simulink library "halout"  (R2021b)
settings: Solver=VariableStepAuto  StartTime=0.0  StopTime=10.0  RelTol=1e-3
undefined symbols (not defined in the file): C_TASK_5MS_S, FALSE, KHAL_CAN1FDAPS3E2E_flg, KHAL_CAN1FDAPS3TxReq_flg, KHAL_CAN1FDVCU2E2E_flg, KHAL_CAN1FDVCU2TxReq_flg, KHAL_CAN1FDVCU3E2E_flg, KHAL_CAN1FDVCU3TxReq_flg, KHAL_CAN1TxReq_flg, KHAL_CAN2TxReq_flg, KHAL_CAN3FDVCU1TxReq_flg, KHAL_CAN3FDVCU2E2E_flg, KHAL_CAN3FDVCU2TxReq_flg, KHAL_CAN3TxReq_flg, KHAL_CAN4FDVCU1E2E_flg, KHAL_CAN4FDVCU1TxReq_flg, KHAL_CAN4TxReq_flg, KHAL_CAN5TxReq_flg, ONE_INT, TRUE, ZERO_INT
libraries: FVT_lib x383, simulink x179
(part 6 of 20)

== system halout/HAL_OUT/CAN2/FD_VCU5_0x245 ==
  BSCP_outputs : Inport  OutDataTypeStr=Bus: BSCP_outputs
  BOUTP_outputs : Inport  Port=2  OutDataTypeStr=Bus: BOUTP_outputs
  EDriveSysErrAccPedalErr : Subsystem
  EDriveSysErrMCUErr : Subsystem
  EDriveSysErrShifterErr : Subsystem
  EDriveSysErrVCUErr : Subsystem
  Ground{,1..6} (7 alike) : Ground
  HVSysErrIsolationErr : Subsystem
  HVSysErrPackErr : Subsystem
  HVSysErrRelayErr : Subsystem
  LVSysErrPwrOutpErr : Subsystem
  LimphomeAct : Subsystem
  LowSOCWarn : Subsystem
  PwrStaErr : Subsystem
  ReVehThdChkSta : Subsystem
  bus_creator : BusCreator  Inputs=12  OutDataTypeStr=Bus: DT_CAN2_SG_FD_VCU5  NonVirtualBus=on
  bus_selector : BusSelector  OutputSignals=VOUTP_EDriveSysErr_VCUErrTmp_flg
  bus_selector1 : BusSelector  OutputSignals=VOUTP_LVSysErrPwrOutErr_flg
  bus_selector2 : BusSelector  OutputSignals=VOUTP_LimpHomeActTmp_flg
  bus_selector3 : BusSelector  OutputSignals=VOUTP_LowSOCWarn_enum
  bus_selector4 : BusSelector  OutputSignals=VOUTP_ReVehThdChkSta_enum
  FD_VCU5 : Outport
  wires:
  BSCP_outputs/1 -> [BSCP_outputs]
  BOUTP_outputs/1 -> [BOUTP_outputs]
  [CAN2_EDriveSysErr_AccPedalErr] -> bus_creator/1  "CAN2_EDriveSysErr_AccPedalErr"
  [CAN2_EDriveSysErr_MCUErr] -> bus_creator/2  "CAN2_EDriveSysErr_MCUErr"
  [CAN2_EDriveSysErr_ShifterErr] -> bus_creator/3  "CAN2_EDriveSysErr_ShifterErr"
  [CAN2_EDriveSysErr_VCUErr] -> bus_creator/4  "CAN2_EDriveSysErr_VCUErr"
  [CAN2_HVSysErr_IsolationErr] -> bus_creator/5  "CAN2_HVSysErr_IsolationErr"
  [CAN2_HVSysErr_PackErr] -> bus_creator/6  "CAN2_HVSysErr_PackErr"
  [CAN2_HVSysErr_RelayErr] -> bus_creator/7  "CAN2_HVSysErr_RelayErr"
  [CAN2_LVSysErr_PwrOutpErr] -> bus_creator/8  "CAN2_LVSysErr_PwrOutpErr"
  [CAN2_LimphomeAct] -> bus_creator/9  "CAN2_LimphomeAct"
  [CAN2_LowSOCWarn] -> bus_creator/10  "CAN2_LowSOCWarn"
  [CAN2_PwrStaErr] -> bus_creator/11  "CAN2_PwrStaErr"
  [CAN2_Re_VehThdChkSta] -> bus_creator/12  "CAN2_Re_VehThdChkSta"
  bus_creator/1 -> FD_VCU5/1
  EDriveSysErrAccPedalErr/1(CAN2_EDriveSysErr_AccPedalErr) -> [CAN2_EDriveSysErr_AccPedalErr]
  EDriveSysErrMCUErr/1(CAN2_EDriveSysErr_MCUErr) -> [CAN2_EDriveSysErr_MCUErr]
  EDriveSysErrShifterErr/1(CAN2_EDriveSysErr_ShifterErr) -> [CAN2_EDriveSysErr_ShifterErr]
  EDriveSysErrVCUErr/1(CAN2_EDriveSysErr_VCUErr) -> [CAN2_EDriveSysErr_VCUErr]
  HVSysErrIsolationErr/1(CAN2_HVSysErr_IsolationErr) -> [CAN2_HVSysErr_IsolationErr]
  HVSysErrPackErr/1(CAN2_HVSysErr_PackErr) -> [CAN2_HVSysErr_PackErr]
  HVSysErrRelayErr/1(CAN2_HVSysErr_RelayErr) -> [CAN2_HVSysErr_RelayErr]
  LVSysErrPwrOutpErr/1(CAN2_LVSysErr_PwrOutpErr) -> [CAN2_LVSysErr_PwrOutpErr]
  LimphomeAct/1(CAN2_LimphomeAct) -> [CAN2_LimphomeAct]
  LowSOCWarn/1(CAN2_LowSOCWarn) -> [CAN2_LowSOCWarn]
  PwrStaErr/1(CAN2_PwrStaErr) -> [CAN2_PwrStaErr]
  ReVehThdChkSta/1(CAN2_Re_VehThdChkSta) -> [CAN2_Re_VehThdChkSta]
  Ground/1 -> EDriveSysErrAccPedalErr/1(EDriveSysErrAccPedalErr)
  Ground1/1 -> EDriveSysErrMCUErr/1(EDriveSysErrMCUErr)
  Ground2/1 -> EDriveSysErrShifterErr/1(EDriveSysErrShifterErr)
  bus_selector/1 -> EDriveSysErrVCUErr/1(EDriveSysErrVCUErr)  "<VOUTP_EDriveSysErr_VCUErrTmp_flg>"
  [BOUTP_outputs] -> bus_selector/1
  Ground3/1 -> HVSysErrIsolationErr/1(HVSysErrIsolationErr)
  Ground4/1 -> HVSysErrPackErr/1(HVSysErrPackErr)
  Ground5/1 -> HVSysErrRelayErr/1(HVSysErrRelayErr)
  bus_selector1/1 -> LVSysErrPwrOutpErr/1(LVSysErrPwrOutpErr)  "<VOUTP_LVSysErrPwrOutErr_flg>"
  [BOUTP_outputs] -> bus_selector1/1
  bus_selector2/1 -> LimphomeAct/1(LimphomeAct)  "<VOUTP_LimpHomeActTmp_flg>"
  [BOUTP_outputs] -> bus_selector2/1
  bus_selector3/1 -> LowSOCWarn/1(LowSOCWarn)  "<VOUTP_LowSOCWarn_enum>"
  [BOUTP_outputs] -> bus_selector3/1
  Ground6/1 -> PwrStaErr/1(PwrStaErr)
  bus_selector4/1 -> ReVehThdChkSta/1(ReVehThdChkSta)  "<VOUTP_ReVehThdChkSta_enum>"
  [BOUTP_outputs] -> bus_selector4/1

== system halout/HAL_OUT/CAN2/FD_VCU6_0x3C3 ==
  BSCP_outputs : Inport  OutDataTypeStr=Bus: BSCP_outputs
  BOUTP_outputs : Inport  Port=2  OutDataTypeStr=Bus: BOUTP_outputs
  FUSIONHWVer1 : Subsystem
  FUSIONHWVer2 : Subsystem
  FUSIONHWVer3 : Subsystem
  FUSIONSWCarModel1 : Subsystem
  FUSIONSWCarModel2 : Subsystem
  FUSIONSWCarModel3 : Subsystem
  FUSIONSWController1 : Subsystem
  FUSIONSWController2 : Subsystem
  FUSIONSWCountry1 : Subsystem
  FUSIONSWCountry2 : Subsystem
  FUSIONSWMajor1 : Subsystem
  FUSIONSWMajor2 : Subsystem
  FUSIONSWMinor1 : Subsystem
  FUSIONSWMinor2 : Subsystem
  FUSIONSWPatch1 : Subsystem
  FUSIONSWPatch2 : Subsystem
  FUSIONSWSHA1 : Subsystem
  FUSIONSWSHA2 : Subsystem
  FUSIONSWSHA3 : Subsystem
  FUSIONSWSHA4 : Subsystem
  FUSIONSWSHA5 : Subsystem
  FUSIONSWSHA6 : Subsystem
  FUSIONSWSHA7 : Subsystem
  FUSIONSWSHA8 : Subsystem
  FUSIONSWVar : Subsystem
  FUSIONSWchange1 : Subsystem
  FUSIONSWchange2 : Subsystem
  FUSIONSWdash1 : Subsystem
  FUSIONSWdash2 : Subsystem
  bus_creator : BusCreator  Inputs=29  OutDataTypeStr=Bus: DT_CAN2_SG_FD_VCU6  NonVirtualBus=on
  bus_selector : BusSelector  OutputSignals=VOUTP_HWVer1_cnt
  bus_selector1 : BusSelector  OutputSignals=VOUTP_HWVer2_cnt
  bus_selector10 : BusSelector  OutputSignals=VOUTP_Major1_cnt
  bus_selector11 : BusSelector  OutputSignals=VOUTP_Major2_cnt
  bus_selector12 : BusSelector  OutputSignals=VOUTP_Minor1_cnt
  bus_selector13 : BusSelector  OutputSignals=VOUTP_Minor2_cnt
  bus_selector14 : BusSelector  OutputSignals=VOUTP_Patch1_cnt
  bus_selector15 : BusSelector  OutputSignals=VOUTP_Patch2_cnt
  bus_selector16 : BusSelector  OutputSignals=VOUTP_SHA1_cnt
  bus_selector17 : BusSelector  OutputSignals=VOUTP_SHA2_cnt
  bus_selector18 : BusSelector  OutputSignals=VOUTP_SHA3_cnt
  bus_selector19 : BusSelector  OutputSignals=VOUTP_SHA4_cnt
  bus_selector2 : BusSelector  OutputSignals=VOUTP_HWVer3_cnt
  bus_selector20 : BusSelector  OutputSignals=VOUTP_SHA5_cnt
  bus_selector21 : BusSelector  OutputSignals=VOUTP_SHA6_cnt
  bus_selector22 : BusSelector  OutputSignals=VOUTP_SHA7_cnt
  bus_selector23 : BusSelector  OutputSignals=VOUTP_SHA8_cnt
  bus_selector24 : BusSelector  OutputSignals=VOUTP_Variation_cnt
  bus_selector25 : BusSelector  OutputSignals=VOUTP_Change1_cnt
  bus_selector26 : BusSelector  OutputSignals=VOUTP_Change2_cnt
  bus_selector27 : BusSelector  OutputSignals=VOUTP_Dash1_cnt
  bus_selector28 : BusSelector  OutputSignals=VOUTP_Dash2_cnt
  bus_selector3 : BusSelector  OutputSignals=VOUTP_CarModel1_cnt
  bus_selector4 : BusSelector  OutputSignals=VOUTP_CarModel2_cnt
  bus_selector5 : BusSelector  OutputSignals=VOUTP_CarModel3_cnt
  bus_selector6 : BusSelector  OutputSignals=VOUTP_ECU1_cnt
  bus_selector7 : BusSelector  OutputSignals=VOUTP_ECU2_cnt
  bus_selector8 : BusSelector  OutputSignals=VOUTP_Country1_cnt
  bus_selector9 : BusSelector  OutputSignals=VOUTP_Country2_cnt
  FD_VCU6 : Outport
  wires:
  BSCP_outputs/1 -> [BSCP_outputs]
  BOUTP_outputs/1 -> [BOUTP_outputs]
  [CAN2_FUSION_HW_Ver1] -> bus_creator/1  "CAN2_FUSION_HW_Ver1"
  [CAN2_FUSION_HW_Ver2] -> bus_creator/2  "CAN2_FUSION_HW_Ver2"
  [CAN2_FUSION_HW_Ver3] -> bus_creator/3  "CAN2_FUSION_HW_Ver3"
  [CAN2_FUSION_SW_CarModel1] -> bus_creator/4  "CAN2_FUSION_SW_CarModel1"
  [CAN2_FUSION_SW_CarModel2] -> bus_creator/5  "CAN2_FUSION_SW_CarModel2"
  [CAN2_FUSION_SW_CarModel3] -> bus_creator/6  "CAN2_FUSION_SW_CarModel3"
  [CAN2_FUSION_SW_Controller1] -> bus_creator/7  "CAN2_FUSION_SW_Controller1"
  [CAN2_FUSION_SW_Controller2] -> bus_creator/8  "CAN2_FUSION_SW_Controller2"
  [CAN2_FUSION_SW_Country1] -> bus_creator/9  "CAN2_FUSION_SW_Country1"
  [CAN2_FUSION_SW_Country2] -> bus_creator/10  "CAN2_FUSION_SW_Country2"
  [CAN2_FUSION_SW_Major1] -> bus_creator/11  "CAN2_FUSION_SW_Major1"
  [CAN2_FUSION_SW_Major2] -> bus_creator/12  "CAN2_FUSION_SW_Major2"
  [CAN2_FUSION_SW_Minor1] -> bus_creator/13  "CAN2_FUSION_SW_Minor1"
  [CAN2_FUSION_SW_Minor2] -> bus_creator/14  "CAN2_FUSION_SW_Minor2"
  [CAN2_FUSION_SW_Patch1] -> bus_creator/15  "CAN2_FUSION_SW_Patch1"
  [CAN2_FUSION_SW_Patch2] -> bus_creator/16  "CAN2_FUSION_SW_Patch2"
  [CAN2_FUSION_SW_SHA1] -> bus_creator/17  "CAN2_FUSION_SW_SHA1"
  [CAN2_FUSION_SW_SHA2] -> bus_creator/18  "CAN2_FUSION_SW_SHA2"
  [CAN2_FUSION_SW_SHA3] -> bus_creator/19  "CAN2_FUSION_SW_SHA3"
  [CAN2_FUSION_SW_SHA4] -> bus_creator/20  "CAN2_FUSION_SW_SHA4"
  [CAN2_FUSION_SW_SHA5] -> bus_creator/21  "CAN2_FUSION_SW_SHA5"
  [CAN2_FUSION_SW_SHA6] -> bus_creator/22  "CAN2_FUSION_SW_SHA6"
  [CAN2_FUSION_SW_SHA7] -> bus_creator/23  "CAN2_FUSION_SW_SHA7"
  [CAN2_FUSION_SW_SHA8] -> bus_creator/24  "CAN2_FUSION_SW_SHA8"
  [CAN2_FUSION_SW_Var] -> bus_creator/25  "CAN2_FUSION_SW_Var"
  [CAN2_FUSION_SW_change1] -> bus_creator/26  "CAN2_FUSION_SW_change1"
  [CAN2_FUSION_SW_change2] -> bus_creator/27  "CAN2_FUSION_SW_change2"
  [CAN2_FUSION_SW_dash1] -> bus_creator/28  "CAN2_FUSION_SW_dash1"
  [CAN2_FUSION_SW_dash2] -> bus_creator/29  "CAN2_FUSION_SW_dash2"
  bus_creator/1 -> FD_VCU6/1
  FUSIONHWVer1/1(CAN2_FUSION_HW_Ver1) -> [CAN2_FUSION_HW_Ver1]
  FUSIONHWVer2/1(CAN2_FUSION_HW_Ver2) -> [CAN2_FUSION_HW_Ver2]
  FUSIONHWVer3/1(CAN2_FUSION_HW_Ver3) -> [CAN2_FUSION_HW_Ver3]
  FUSIONSWCarModel1/1(CAN2_FUSION_SW_CarModel1) -> [CAN2_FUSION_SW_CarModel1]
  FUSIONSWCarModel2/1(CAN2_FUSION_SW_CarModel2) -> [CAN2_FUSION_SW_CarModel2]
  FUSIONSWCarModel3/1(CAN2_FUSION_SW_CarModel3) -> [CAN2_FUSION_SW_CarModel3]
  FUSIONSWController1/1(CAN2_FUSION_SW_Controller1) -> [CAN2_FUSION_SW_Controller1]
  FUSIONSWController2/1(CAN2_FUSION_SW_Controller2) -> [CAN2_FUSION_SW_Controller2]
  FUSIONSWCountry1/1(CAN2_FUSION_SW_Country1) -> [CAN2_FUSION_SW_Country1]
  FUSIONSWCountry2/1(CAN2_FUSION_SW_Country2) -> [CAN2_FUSION_SW_Country2]
  FUSIONSWMajor1/1(CAN2_FUSION_SW_Major1) -> [CAN2_FUSION_SW_Major1]
  FUSIONSWMajor2/1(CAN2_FUSION_SW_Major2) -> [CAN2_FUSION_SW_Major2]
  FUSIONSWMinor1/1(CAN2_FUSION_SW_Minor1) -> [CAN2_FUSION_SW_Minor1]
  FUSIONSWMinor2/1(CAN2_FUSION_SW_Minor2) -> [CAN2_FUSION_SW_Minor2]
  FUSIONSWPatch1/1(CAN2_FUSION_SW_Patch1) -> [CAN2_FUSION_SW_Patch1]
  FUSIONSWPatch2/1(CAN2_FUSION_SW_Patch2) -> [CAN2_FUSION_SW_Patch2]
  FUSIONSWSHA1/1(CAN2_FUSION_SW_SHA1) -> [CAN2_FUSION_SW_SHA1]
  FUSIONSWSHA2/1(CAN2_FUSION_SW_SHA2) -> [CAN2_FUSION_SW_SHA2]
  FUSIONSWSHA3/1(CAN2_FUSION_SW_SHA3) -> [CAN2_FUSION_SW_SHA3]
  FUSIONSWSHA4/1(CAN2_FUSION_SW_SHA4) -> [CAN2_FUSION_SW_SHA4]
  FUSIONSWSHA5/1(CAN2_FUSION_SW_SHA5) -> [CAN2_FUSION_SW_SHA5]
  FUSIONSWSHA6/1(CAN2_FUSION_SW_SHA6) -> [CAN2_FUSION_SW_SHA6]
  FUSIONSWSHA7/1(CAN2_FUSION_SW_SHA7) -> [CAN2_FUSION_SW_SHA7]
  FUSIONSWSHA8/1(CAN2_FUSION_SW_SHA8) -> [CAN2_FUSION_SW_SHA8]
  FUSIONSWVar/1(CAN2_FUSION_SW_Var) -> [CAN2_FUSION_SW_Var]
  FUSIONSWchange1/1(CAN2_FUSION_SW_change1) -> [CAN2_FUSION_SW_change1]
  FUSIONSWchange2/1(CAN2_FUSION_SW_change2) -> [CAN2_FUSION_SW_change2]
  FUSIONSWdash1/1(CAN2_FUSION_SW_dash1) -> [CAN2_FUSION_SW_dash1]
  FUSIONSWdash2/1(CAN2_FUSION_SW_dash2) -> [CAN2_FUSION_SW_dash2]
  bus_selector/1 -> FUSIONHWVer1/1(FUSIONHWVer1)  "<VOUTP_HWVer1_cnt>"
  [BOUTP_outputs] -> bus_selector/1
  bus_selector1/1 -> FUSIONHWVer2/1(FUSIONHWVer2)  "<VOUTP_HWVer2_cnt>"
  [BOUTP_outputs] -> bus_selector1/1
  bus_selector2/1 -> FUSIONHWVer3/1(FUSIONHWVer3)  "<VOUTP_HWVer3_cnt>"
  [BOUTP_outputs] -> bus_selector2/1
  bus_selector3/1 -> FUSIONSWCarModel1/1(FUSIONSWCarModel1)  "<VOUTP_CarModel1_cnt>"
  [BOUTP_outputs] -> bus_selector3/1
  bus_selector4/1 -> FUSIONSWCarModel2/1(FUSIONSWCarModel2)  "<VOUTP_CarModel2_cnt>"
  [BOUTP_outputs] -> bus_selector4/1
  bus_selector5/1 -> FUSIONSWCarModel3/1(FUSIONSWCarModel3)  "<VOUTP_CarModel3_cnt>"
  [BOUTP_outputs] -> bus_selector5/1
  bus_selector6/1 -> FUSIONSWController1/1(FUSIONSWController1)  "<VOUTP_ECU1_cnt>"
  [BOUTP_outputs] -> bus_selector6/1
  bus_selector7/1 -> FUSIONSWController2/1(FUSIONSWController2)  "<VOUTP_ECU2_cnt>"
  [BOUTP_outputs] -> bus_selector7/1
  bus_selector8/1 -> FUSIONSWCountry1/1(FUSIONSWCountry1)  "<VOUTP_Country1_cnt>"
  [BOUTP_outputs] -> bus_selector8/1
  bus_selector9/1 -> FUSIONSWCountry2/1(FUSIONSWCountry2)  "<VOUTP_Country2_cnt>"
  [BOUTP_outputs] -> bus_selector9/1
  bus_selector10/1 -> FUSIONSWMajor1/1(FUSIONSWMajor1)  "<VOUTP_Major1_cnt>"
  [BOUTP_outputs] -> bus_selector10/1
  bus_selector11/1 -> FUSIONSWMajor2/1(FUSIONSWMajor2)  "<VOUTP_Major2_cnt>"
  [BOUTP_outputs] -> bus_selector11/1
  bus_selector12/1 -> FUSIONSWMinor1/1(FUSIONSWMinor1)  "<VOUTP_Minor1_cnt>"
  [BOUTP_outputs] -> bus_selector12/1
  bus_selector13/1 -> FUSIONSWMinor2/1(FUSIONSWMinor2)  "<VOUTP_Minor2_cnt>"
  [BOUTP_outputs] -> bus_selector13/1
  bus_selector14/1 -> FUSIONSWPatch1/1(FUSIONSWPatch1)  "<VOUTP_Patch1_cnt>"
  [BOUTP_outputs] -> bus_selector14/1
  bus_selector15/1 -> FUSIONSWPatch2/1(FUSIONSWPatch2)  "<VOUTP_Patch2_cnt>"
  [BOUTP_outputs] -> bus_selector15/1
  bus_selector16/1 -> FUSIONSWSHA1/1(FUSIONSWSHA1)  "<VOUTP_SHA1_cnt>"
  [BOUTP_outputs] -> bus_selector16/1
  bus_selector17/1 -> FUSIONSWSHA2/1(FUSIONSWSHA2)  "<VOUTP_SHA2_cnt>"
  [BOUTP_outputs] -> bus_selector17/1
  bus_selector18/1 -> FUSIONSWSHA3/1(FUSIONSWSHA3)  "<VOUTP_SHA3_cnt>"
  [BOUTP_outputs] -> bus_selector18/1
  bus_selector19/1 -> FUSIONSWSHA4/1(FUSIONSWSHA4)  "<VOUTP_SHA4_cnt>"
  [BOUTP_outputs] -> bus_selector19/1
  bus_selector20/1 -> FUSIONSWSHA5/1(FUSIONSWSHA5)  "<VOUTP_SHA5_cnt>"
  [BOUTP_outputs] -> bus_selector20/1
  bus_selector21/1 -> FUSIONSWSHA6/1(FUSIONSWSHA6)  "<VOUTP_SHA6_cnt>"
  [BOUTP_outputs] -> bus_selector21/1
  bus_selector22/1 -> FUSIONSWSHA7/1(FUSIONSWSHA7)  "<VOUTP_SHA7_cnt>"
  [BOUTP_outputs] -> bus_selector22/1
  bus_selector23/1 -> FUSIONSWSHA8/1(FUSIONSWSHA8)  "<VOUTP_SHA8_cnt>"
  [BOUTP_outputs] -> bus_selector23/1
  bus_selector24/1 -> FUSIONSWVar/1(FUSIONSWVar)  "<VOUTP_Variation_cnt>"
  [BOUTP_outputs] -> bus_selector24/1
  bus_selector25/1 -> FUSIONSWchange1/1(FUSIONSWchange1)  "<VOUTP_Change1_cnt>"
  [BOUTP_outputs] -> bus_selector25/1
  bus_selector26/1 -> FUSIONSWchange2/1(FUSIONSWchange2)  "<VOUTP_Change2_cnt>"
  [BOUTP_outputs] -> bus_selector26/1
  bus_selector27/1 -> FUSIONSWdash1/1(FUSIONSWdash1)  "<VOUTP_Dash1_cnt>"
  [BOUTP_outputs] -> bus_selector27/1
  bus_selector28/1 -> FUSIONSWdash2/1(FUSIONSWdash2)  "<VOUTP_Dash2_cnt>"
  [BOUTP_outputs] -> bus_selector28/1

== system halout/HAL_OUT/CAN2/FD_VMC1_0x17F ==
  BSCP_outputs : Inport  OutDataTypeStr=Bus: BSCP_outputs
  BOUTP_outputs : Inport  Port=2  OutDataTypeStr=Bus: BOUTP_outputs
  CCMSASpdWar : Subsystem
  bus_creator : BusCreator  Inputs=1  OutDataTypeStr=Bus: DT_CAN2_SG_FD_VMC1  NonVirtualBus=on
  bus_selector : BusSelector  OutputSignals=VOUTP_CCMSASpdWar_flg
  FD_VMC1 : Outport
  wires:
  BSCP_outputs/1 -> [BSCP_outputs]
  BOUTP_outputs/1 -> [BOUTP_outputs]
  [CAN2_CCMSA_SpdWar] -> bus_creator/1  "CAN2_CCMSA_SpdWar"
  bus_creator/1 -> FD_VMC1/1
  CCMSASpdWar/1(CAN2_CCMSA_SpdWar) -> [CAN2_CCMSA_SpdWar]
  bus_selector/1 -> CCMSASpdWar/1(CCMSASpdWar)  "<VOUTP_CCMSASpdWar_flg>"
  [BOUTP_outputs] -> bus_selector/1

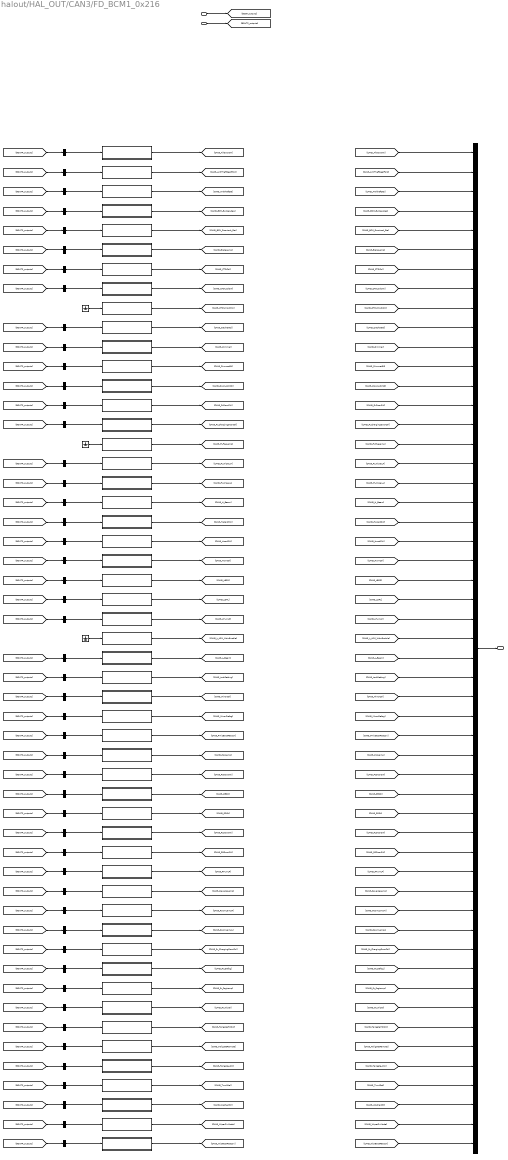
== system halout/HAL_OUT/CAN3/FD_BCM1_0x216 ==
  BSCP_outputs : Inport  OutDataTypeStr=Bus: BSCP_outputs
  BOUTP_outputs : Inport  Port=2  OutDataTypeStr=Bus: BOUTP_outputs
  AllDoorSW : Subsystem
  AntiTheftSeatFold : Subsystem
  AntitheftSta : Subsystem
  BCMBuzzerReq : Subsystem
  BCMDoorLockSta : Subsystem
  BrakeLamp : Subsystem
  CTDCtrl : Subsystem
  CTDLockSW : Subsystem
  CTDUnlockSW : Subsystem
  CrashDetd : Subsystem
  Dimmer : Subsystem
  DimmerEN : Subsystem
  DoorLockIND : Subsystem
  DrDoorSW : Subsystem
  FrChargingDoorCtrl : Subsystem
  FrFogLamp : Subsystem
  FrWiperH : Subsystem
  FrWiperL : Subsystem
  Ground : Ground
  Ground1 : Ground
  Ground2 : Ground
  HBeam : Subsystem
  HazardSW : Subsystem
  HoodSW : Subsystem
  HornCtrl : Subsystem
  LAPMWdwEnable : Subsystem
  LBSD : Subsystem
  LBeam : Subsystem
  LDRL : Subsystem
  LTurnLP : Subsystem
  LockSetting : Subsystem
  MirrorCtrl : Subsystem
  MirrorDefog : Subsystem
  PmicBootReason : Subsystem
  PosLamp : Subsystem
  PsDoorSW : Subsystem
  RBSD : Subsystem
  RDRL : Subsystem
  RLDoorSW : Subsystem
  RRDoorSW : Subsystem
  RTurnLP : Subsystem
  ReverseLamp : Subsystem
  RoomLampH : Subsystem
  RoomLampL : Subsystem
  RrChargingDoorCtrl : Subsystem
  RrDefog : Subsystem
  RrFogLamp : Subsystem
  RrWiper : Subsystem
  TailgateHDSW : Subsystem
  TailgateRemote : Subsystem
  TailgateSW : Subsystem
  TrunkRel : Subsystem
  WasherCtrl : Subsystem
  WiperFixMode : Subsystem
  WisrBootReason : Subsystem
  bus_creator : BusCreator  Inputs=52  OutDataTypeStr=Bus: DT_CAN3_SG_FD_BCM1  NonVirtualBus=on
  bus_selector : BusSelector  OutputSignals=VOUTP_AllDoorSW_flg
  bus_selector1 : BusSelector  OutputSignals=VOUTP_AntitheftSeatFlod_flg
  bus_selector10 : BusSelector  OutputSignals=VOUTP_DimmerEN_flg
  bus_selector11 : BusSelector  OutputSignals=VOUTP_DoorLockIND_flg
  bus_selector12 : BusSelector  OutputSignals=VOUTP_DrDoorSW_flg
  bus_selector13 : BusSelector  OutputSignals=VOUTP_FrChargingDoorCtrl_enum
  bus_selector14 : BusSelector  OutputSignals=VOUTP_FrWiperH_flg
  bus_selector15 : BusSelector  OutputSignals=VOUTP_FrWiperL_flg
  bus_selector16 : BusSelector  OutputSignals=VOUTP_HBeam_flg
  bus_selector17 : BusSelector  OutputSignals=VOUTP_HazardSW_flg
  bus_selector18 : BusSelector  OutputSignals=VOUTP_HoodSW_flg
  bus_selector19 : BusSelector  OutputSignals=VOUTP_HornCtrl_flg
  bus_selector2 : BusSelector  OutputSignals=VOUTP_AntitheftSta_enum
  bus_selector20 : BusSelector  OutputSignals=VOUTP_LBSD_flg
  bus_selector21 : BusSelector  OutputSignals=VOUTP_LDRL_flg
  bus_selector22 : BusSelector  OutputSignals=VOUTP_LTurnLP_flg
  bus_selector23 : BusSelector  OutputSignals=VOUTP_LBeam_flg
  bus_selector24 : BusSelector  OutputSignals=VOUTP_LockSetting_flg
  bus_selector25 : BusSelector  OutputSignals=VOUTP_MirrorCtrl_enum
  bus_selector26 : BusSelector  OutputSignals=VOUTP_MirrorDefog_flg
  bus_selector27 : BusSelector  OutputSignals=VOUTP_PmicBootReason_enum
  bus_selector28 : BusSelector  OutputSignals=VOUTP_PosLamp_flg
  bus_selector29 : BusSelector  OutputSignals=VOUTP_PsDoorSW_flg
  bus_selector3 : BusSelector  OutputSignals=VOUTP_BCMBuzzerReq_flg
  bus_selector30 : BusSelector  OutputSignals=VOUTP_RBSD_flg
  bus_selector31 : BusSelector  OutputSignals=VOUTP_RDRL_flg
  bus_selector32 : BusSelector  OutputSignals=VOUTP_RLDoorSW_flg
  bus_selector33 : BusSelector  OutputSignals=VOUTP_RRDoorSW_flg
  bus_selector34 : BusSelector  OutputSignals=VOUTP_RTurnLP_flg
  bus_selector35 : BusSelector  OutputSignals=VOUTP_ReverseLamp_flg
  bus_selector36 : BusSelector  OutputSignals=VOUTP_RoomLampH_flg
  bus_selector37 : BusSelector  OutputSignals=VOUTP_RoomLampL_flg
  bus_selector38 : BusSelector  OutputSignals=VOUTP_RrChargingDoorCtrl_enum
  bus_selector39 : BusSelector  OutputSignals=VOUTP_RrDefog_flg
  bus_selector4 : BusSelector  OutputSignals=VOUTP_BCMDoorLockSta_flg
  bus_selector40 : BusSelector  OutputSignals=VOUTP_RrFogLamp_flg
  bus_selector41 : BusSelector  OutputSignals=VOUTP_RrWiper_flg
  bus_selector42 : BusSelector  OutputSignals=VOUTP_TailgateHDSW_flg
  bus_selector43 : BusSelector  OutputSignals=VOUTP_TailgateRemote_enum
  bus_selector44 : BusSelector  OutputSignals=VOUTP_TailgateSW_flg
  bus_selector45 : BusSelector  OutputSignals=VOUTP_TrunkRel_flg
  bus_selector46 : BusSelector  OutputSignals=VOUTP_WasherCtrl_enum
  bus_selector47 : BusSelector  OutputSignals=VOUTP_WiperFixMode_flg
  bus_selector48 : BusSelector  OutputSignals=VOUTP_WisrBootReason_raw32
  bus_selector5 : BusSelector  OutputSignals=VOUTP_BrakeLamp_flg
  bus_selector6 : BusSelector  OutputSignals=VOUTP_CTDCtrl_enum
  bus_selector7 : BusSelector  OutputSignals=VOUTP_CTDLockSW_flg
  bus_selector8 : BusSelector  OutputSignals=VOUTP_CrashDetd_flg
  bus_selector9 : BusSelector  OutputSignals=VOUTP_Dimmer_pct
  FD_BCM1 : Outport
  wires:
  BSCP_outputs/1 -> [BSCP_outputs]
  BOUTP_outputs/1 -> [BOUTP_outputs]
  [CAN3_AllDoorSW] -> bus_creator/1  "CAN3_AllDoorSW"
  [CAN3_AntiTheftSeatFold] -> bus_creator/2  "CAN3_AntiTheftSeatFold"
  [CAN3_AntitheftSta] -> bus_creator/3  "CAN3_AntitheftSta"
  [CAN3_BCM_Buzzer_Req] -> bus_creator/4  "CAN3_BCM_Buzzer_Req"
  [CAN3_BCM_DoorLock_Sta] -> bus_creator/5  "CAN3_BCM_DoorLock_Sta"
  [CAN3_BrakeLamp] -> bus_creator/6  "CAN3_BrakeLamp"
  [CAN3_CTDCtrl] -> bus_creator/7  "CAN3_CTDCtrl"
  [CAN3_CTDLockSW] -> bus_creator/8  "CAN3_CTDLockSW"
  [CAN3_CTDUnlockSW] -> bus_creator/9  "CAN3_CTDUnlockSW"
  [CAN3_CrashDetd] -> bus_creator/10  "CAN3_CrashDetd"
  [CAN3_Dimmer] -> bus_creator/11  "CAN3_Dimmer"
  [CAN3_DimmerEN] -> bus_creator/12  "CAN3_DimmerEN"
  [CAN3_DoorLockIND] -> bus_creator/13  "CAN3_DoorLockIND"
  [CAN3_DrDoorSW] -> bus_creator/14  "CAN3_DrDoorSW"
  [CAN3_Fr_ChargingDoorCtrl] -> bus_creator/15  "CAN3_Fr_ChargingDoorCtrl"
  [CAN3_Fr_FogLamp] -> bus_creator/16  "CAN3_Fr_FogLamp"
  [CAN3_Fr_Wiper_H] -> bus_creator/17  "CAN3_Fr_Wiper_H"
  [CAN3_Fr_Wiper_L] -> bus_creator/18  "CAN3_Fr_Wiper_L"
  [CAN3_H_Beam] -> bus_creator/19  "CAN3_H_Beam"
  [CAN3_HazardSW] -> bus_creator/20  "CAN3_HazardSW"
  [CAN3_HoodSW] -> bus_creator/21  "CAN3_HoodSW"
  [CAN3_HornCtrl] -> bus_creator/22  "CAN3_HornCtrl"
  [CAN3_LBSD] -> bus_creator/23  "CAN3_LBSD"
  [CAN3_LDRL] -> bus_creator/24  "CAN3_LDRL"
  [CAN3_LTurnLP] -> bus_creator/25  "CAN3_LTurnLP"
  [CAN3_L_APM_WdwEnable] -> bus_creator/26  "CAN3_L_APM_WdwEnable"
  [CAN3_L_Beam] -> bus_creator/27  "CAN3_L_Beam"
  [CAN3_LockSetting] -> bus_creator/28  "CAN3_LockSetting"
  [CAN3_MirrorCtrl] -> bus_creator/29  "CAN3_MirrorCtrl"
  [CAN3_MirrorDefog] -> bus_creator/30  "CAN3_MirrorDefog"
  [CAN3_PmicBootReason] -> bus_creator/31  "CAN3_PmicBootReason"
  [CAN3_PosLamp] -> bus_creator/32  "CAN3_PosLamp"
  [CAN3_PsDoorSW] -> bus_creator/33  "CAN3_PsDoorSW"
  [CAN3_RBSD] -> bus_creator/34  "CAN3_RBSD"
  [CAN3_RDRL] -> bus_creator/35  "CAN3_RDRL"
  [CAN3_RLDoorSW] -> bus_creator/36  "CAN3_RLDoorSW"
  [CAN3_RRDoorSW] -> bus_creator/37  "CAN3_RRDoorSW"
  [CAN3_RTurnLP] -> bus_creator/38  "CAN3_RTurnLP"
  [CAN3_ReverseLamp] -> bus_creator/39  "CAN3_ReverseLamp"
  [CAN3_RoomLampH] -> bus_creator/40  "CAN3_RoomLampH"
  [CAN3_RoomLampL] -> bus_creator/41  "CAN3_RoomLampL"
  [CAN3_Rr_ChargingDoorCtrl] -> bus_creator/42  "CAN3_Rr_ChargingDoorCtrl"
  [CAN3_Rr_Defog] -> bus_creator/43  "CAN3_Rr_Defog"
  [CAN3_Rr_FogLamp] -> bus_creator/44  "CAN3_Rr_FogLamp"
  [CAN3_Rr_Wiper] -> bus_creator/45  "CAN3_Rr_Wiper"
  [CAN3_TailgateHDSW] -> bus_creator/46  "CAN3_TailgateHDSW"
  [CAN3_TailgateRemote] -> bus_creator/47  "CAN3_TailgateRemote"
  [CAN3_Tailgate_SW] -> bus_creator/48  "CAN3_Tailgate_SW"
  [CAN3_TrunkRel] -> bus_creator/49  "CAN3_TrunkRel"
  [CAN3_WasherCtrl] -> bus_creator/50  "CAN3_WasherCtrl"
  [CAN3_WiperFixMode] -> bus_creator/51  "CAN3_WiperFixMode"
  [CAN3_WisrBootReason] -> bus_creator/52  "CAN3_WisrBootReason"
  bus_creator/1 -> FD_BCM1/1
  AllDoorSW/1(CAN3_AllDoorSW) -> [CAN3_AllDoorSW]
  AntiTheftSeatFold/1(CAN3_AntiTheftSeatFold) -> [CAN3_AntiTheftSeatFold]
  AntitheftSta/1(CAN3_AntitheftSta) -> [CAN3_AntitheftSta]
  BCMBuzzerReq/1(CAN3_BCM_Buzzer_Req) -> [CAN3_BCM_Buzzer_Req]
  BCMDoorLockSta/1(CAN3_BCM_DoorLock_Sta) -> [CAN3_BCM_DoorLock_Sta]
  BrakeLamp/1(CAN3_BrakeLamp) -> [CAN3_BrakeLamp]
  CTDCtrl/1(CAN3_CTDCtrl) -> [CAN3_CTDCtrl]
  CTDLockSW/1(CAN3_CTDLockSW) -> [CAN3_CTDLockSW]
  CTDUnlockSW/1(CAN3_CTDUnlockSW) -> [CAN3_CTDUnlockSW]
  CrashDetd/1(CAN3_CrashDetd) -> [CAN3_CrashDetd]
  Dimmer/1(CAN3_Dimmer) -> [CAN3_Dimmer]
  DimmerEN/1(CAN3_DimmerEN) -> [CAN3_DimmerEN]
  DoorLockIND/1(CAN3_DoorLockIND) -> [CAN3_DoorLockIND]
  DrDoorSW/1(CAN3_DrDoorSW) -> [CAN3_DrDoorSW]
  FrChargingDoorCtrl/1(CAN3_Fr_ChargingDoorCtrl) -> [CAN3_Fr_ChargingDoorCtrl]
  FrFogLamp/1(CAN3_Fr_FogLamp) -> [CAN3_Fr_FogLamp]
  FrWiperH/1(CAN3_Fr_Wiper_H) -> [CAN3_Fr_Wiper_H]
  FrWiperL/1(CAN3_Fr_Wiper_L) -> [CAN3_Fr_Wiper_L]
  HBeam/1(CAN3_H_Beam) -> [CAN3_H_Beam]
  HazardSW/1(CAN3_HazardSW) -> [CAN3_HazardSW]
  HoodSW/1(CAN3_HoodSW) -> [CAN3_HoodSW]
  HornCtrl/1(CAN3_HornCtrl) -> [CAN3_HornCtrl]
  LBSD/1(CAN3_LBSD) -> [CAN3_LBSD]
  LDRL/1(CAN3_LDRL) -> [CAN3_LDRL]
  LTurnLP/1(CAN3_LTurnLP) -> [CAN3_LTurnLP]
  LAPMWdwEnable/1(CAN3_L_APM_WdwEnable) -> [CAN3_L_APM_WdwEnable]
  LBeam/1(CAN3_L_Beam) -> [CAN3_L_Beam]
  LockSetting/1(CAN3_LockSetting) -> [CAN3_LockSetting]
  MirrorCtrl/1(CAN3_MirrorCtrl) -> [CAN3_MirrorCtrl]
  MirrorDefog/1(CAN3_MirrorDefog) -> [CAN3_MirrorDefog]
  PmicBootReason/1(CAN3_PmicBootReason) -> [CAN3_PmicBootReason]
  PosLamp/1(CAN3_PosLamp) -> [CAN3_PosLamp]
  PsDoorSW/1(CAN3_PsDoorSW) -> [CAN3_PsDoorSW]
  RBSD/1(CAN3_RBSD) -> [CAN3_RBSD]
  RDRL/1(CAN3_RDRL) -> [CAN3_RDRL]
  RLDoorSW/1(CAN3_RLDoorSW) -> [CAN3_RLDoorSW]
  RRDoorSW/1(CAN3_RRDoorSW) -> [CAN3_RRDoorSW]
  RTurnLP/1(CAN3_RTurnLP) -> [CAN3_RTurnLP]
  ReverseLamp/1(CAN3_ReverseLamp) -> [CAN3_ReverseLamp]
  RoomLampH/1(CAN3_RoomLampH) -> [CAN3_RoomLampH]
  RoomLampL/1(CAN3_RoomLampL) -> [CAN3_RoomLampL]
  RrChargingDoorCtrl/1(CAN3_Rr_ChargingDoorCtrl) -> [CAN3_Rr_ChargingDoorCtrl]
  RrDefog/1(CAN3_Rr_Defog) -> [CAN3_Rr_Defog]
  RrFogLamp/1(CAN3_Rr_FogLamp) -> [CAN3_Rr_FogLamp]
  RrWiper/1(CAN3_Rr_Wiper) -> [CAN3_Rr_Wiper]
  TailgateHDSW/1(CAN3_TailgateHDSW) -> [CAN3_TailgateHDSW]
  TailgateRemote/1(CAN3_TailgateRemote) -> [CAN3_TailgateRemote]
  TailgateSW/1(CAN3_Tailgate_SW) -> [CAN3_Tailgate_SW]
  TrunkRel/1(CAN3_TrunkRel) -> [CAN3_TrunkRel]
  WasherCtrl/1(CAN3_WasherCtrl) -> [CAN3_WasherCtrl]
  WiperFixMode/1(CAN3_WiperFixMode) -> [CAN3_WiperFixMode]
  WisrBootReason/1(CAN3_WisrBootReason) -> [CAN3_WisrBootReason]
  bus_selector/1 -> AllDoorSW/1(AllDoorSW)  "<VOUTP_AllDoorSW_flg>"
  [BOUTP_outputs] -> bus_selector/1
  bus_selector1/1 -> AntiTheftSeatFold/1(AntiTheftSeatFold)  "<VOUTP_AntitheftSeatFlod_flg>"
  [BOUTP_outputs] -> bus_selector1/1
  bus_selector2/1 -> AntitheftSta/1(AntitheftSta)  "<VOUTP_AntitheftSta_enum>"
  [BOUTP_outputs] -> bus_selector2/1
  bus_selector3/1 -> BCMBuzzerReq/1(BCMBuzzerReq)  "<VOUTP_BCMBuzzerReq_flg>"
  [BOUTP_outputs] -> bus_selector3/1
  bus_selector4/1 -> BCMDoorLockSta/1(BCMDoorLockSta)  "<VOUTP_BCMDoorLockSta_flg>"
  [BOUTP_outputs] -> bus_selector4/1
  bus_selector5/1 -> BrakeLamp/1(BrakeLamp)  "<VOUTP_BrakeLamp_flg>"
  [BOUTP_outputs] -> bus_selector5/1
  bus_selector6/1 -> CTDCtrl/1(CTDCtrl)  "<VOUTP_CTDCtrl_enum>"
  [BOUTP_outputs] -> bus_selector6/1
  bus_selector7/1 -> CTDLockSW/1(CTDLockSW)  "<VOUTP_CTDLockSW_flg>"
  [BOUTP_outputs] -> bus_selector7/1
  Ground/1 -> CTDUnlockSW/1(CTDUnlockSW)
  bus_selector8/1 -> CrashDetd/1(CrashDetd)  "<VOUTP_CrashDetd_flg>"
  [BOUTP_outputs] -> bus_selector8/1
  bus_selector9/1 -> Dimmer/1(Dimmer)  "<VOUTP_Dimmer_pct>"
  [BOUTP_outputs] -> bus_selector9/1
  bus_selector10/1 -> DimmerEN/1(DimmerEN)  "<VOUTP_DimmerEN_flg>"
  [BOUTP_outputs] -> bus_selector10/1
  bus_selector11/1 -> DoorLockIND/1(DoorLockIND)  "<VOUTP_DoorLockIND_flg>"
  [BOUTP_outputs] -> bus_selector11/1
  bus_selector12/1 -> DrDoorSW/1(DrDoorSW)  "<VOUTP_DrDoorSW_flg>"
  [BOUTP_outputs] -> bus_selector12/1
  bus_selector13/1 -> FrChargingDoorCtrl/1(FrChargingDoorCtrl)  "<VOUTP_FrChargingDoorCtrl_enum>"
  [BOUTP_outputs] -> bus_selector13/1
  Ground1/1 -> FrFogLamp/1(FrFogLamp)
  bus_selector14/1 -> FrWiperH/1(FrWiperH)  "<VOUTP_FrWiperH_flg>"
  [BOUTP_outputs] -> bus_selector14/1
  bus_selector15/1 -> FrWiperL/1(FrWiperL)  "<VOUTP_FrWiperL_flg>"
  [BOUTP_outputs] -> bus_selector15/1
  bus_selector16/1 -> HBeam/1(HBeam)  "<VOUTP_HBeam_flg>"
  [BOUTP_outputs] -> bus_selector16/1
  bus_selector17/1 -> HazardSW/1(HazardSW)  "<VOUTP_HazardSW_flg>"
  [BOUTP_outputs] -> bus_selector17/1
  bus_selector18/1 -> HoodSW/1(HoodSW)  "<VOUTP_HoodSW_flg>"
  [BOUTP_outputs] -> bus_selector18/1
  bus_selector19/1 -> HornCtrl/1(HornCtrl)  "<VOUTP_HornCtrl_flg>"
  [BOUTP_outputs] -> bus_selector19/1
  bus_selector20/1 -> LBSD/1(LBSD)  "<VOUTP_LBSD_flg>"
  [BOUTP_outputs] -> bus_selector20/1
  bus_selector21/1 -> LDRL/1(LDRL)  "<VOUTP_LDRL_flg>"
  [BOUTP_outputs] -> bus_selector21/1
  bus_selector22/1 -> LTurnLP/1(LTurnLP)  "<VOUTP_LTurnLP_flg>"
  [BOUTP_outputs] -> bus_selector22/1
  Ground2/1 -> LAPMWdwEnable/1(LAPMWdwEnable)
  bus_selector23/1 -> LBeam/1(LBeam)  "<VOUTP_LBeam_flg>"
  [BOUTP_outputs] -> bus_selector23/1
  bus_selector24/1 -> LockSetting/1(LockSetting)  "<VOUTP_LockSetting_flg>"
  [BOUTP_outputs] -> bus_selector24/1
  bus_selector25/1 -> MirrorCtrl/1(MirrorCtrl)  "<VOUTP_MirrorCtrl_enum>"
  [BOUTP_outputs] -> bus_selector25/1
  bus_selector26/1 -> MirrorDefog/1(MirrorDefog)  "<VOUTP_MirrorDefog_flg>"
  [BOUTP_outputs] -> bus_selector26/1
  bus_selector27/1 -> PmicBootReason/1(PmicBootReason)  "<VOUTP_PmicBootReason_enum>"
  [BOUTP_outputs] -> bus_selector27/1
  bus_selector28/1 -> PosLamp/1(PosLamp)  "<VOUTP_PosLamp_flg>"
  [BOUTP_outputs] -> bus_selector28/1
  bus_selector29/1 -> PsDoorSW/1(PsDoorSW)  "<VOUTP_PsDoorSW_flg>"
  [BOUTP_outputs] -> bus_selector29/1
  bus_selector30/1 -> RBSD/1(RBSD)  "<VOUTP_RBSD_flg>"
  [BOUTP_outputs] -> bus_selector30/1
  bus_selector31/1 -> RDRL/1(RDRL)  "<VOUTP_RDRL_flg>"
  [BOUTP_outputs] -> bus_selector31/1
  bus_selector32/1 -> RLDoorSW/1(RLDoorSW)  "<VOUTP_RLDoorSW_flg>"
  [BOUTP_outputs] -> bus_selector32/1
  bus_selector33/1 -> RRDoorSW/1(RRDoorSW)  "<VOUTP_RRDoorSW_flg>"
  [BOUTP_outputs] -> bus_selector33/1
  bus_selector34/1 -> RTurnLP/1(RTurnLP)  "<VOUTP_RTurnLP_flg>"
  [BOUTP_outputs] -> bus_selector34/1
  bus_selector35/1 -> ReverseLamp/1(ReverseLamp)  "<VOUTP_ReverseLamp_flg>"
  [BOUTP_outputs] -> bus_selector35/1
  bus_selector36/1 -> RoomLampH/1(RoomLampH)  "<VOUTP_RoomLampH_flg>"
  [BOUTP_outputs] -> bus_selector36/1
  bus_selector37/1 -> RoomLampL/1(RoomLampL)  "<VOUTP_RoomLampL_flg>"
  [BOUTP_outputs] -> bus_selector37/1
  bus_selector38/1 -> RrChargingDoorCtrl/1(RrChargingDoorCtrl)  "<VOUTP_RrChargingDoorCtrl_enum>"
  [BOUTP_outputs] -> bus_selector38/1
  bus_selector39/1 -> RrDefog/1(RrDefog)  "<VOUTP_RrDefog_flg>"
  [BOUTP_outputs] -> bus_selector39/1
  bus_selector40/1 -> RrFogLamp/1(RrFogLamp)  "<VOUTP_RrFogLamp_flg>"
  [BOUTP_outputs] -> bus_selector40/1
  bus_selector41/1 -> RrWiper/1(RrWiper)  "<VOUTP_RrWiper_flg>"
  [BOUTP_outputs] -> bus_selector41/1
  bus_selector42/1 -> TailgateHDSW/1(TailgateHDSW)  "<VOUTP_TailgateHDSW_flg>"
  [BOUTP_outputs] -> bus_selector42/1
  bus_selector43/1 -> TailgateRemote/1(TailgateRemote)  "<VOUTP_TailgateRemote_enum>"
  [BOUTP_outputs] -> bus_selector43/1
  bus_selector44/1 -> TailgateSW/1(TailgateSW)  "<VOUTP_TailgateSW_flg>"
  [BOUTP_outputs] -> bus_selector44/1
  bus_selector45/1 -> TrunkRel/1(TrunkRel)  "<VOUTP_TrunkRel_flg>"
  [BOUTP_outputs] -> bus_selector45/1
  bus_selector46/1 -> WasherCtrl/1(WasherCtrl)  "<VOUTP_WasherCtrl_enum>"
  [BOUTP_outputs] -> bus_selector46/1
  bus_selector47/1 -> WiperFixMode/1(WiperFixMode)  "<VOUTP_WiperFixMode_flg>"
  [BOUTP_outputs] -> bus_selector47/1
  bus_selector48/1 -> WisrBootReason/1(WisrBootReason)  "<VOUTP_WisrBootReason_raw32>"
  [BOUTP_outputs] -> bus_selector48/1

== system halout/HAL_OUT/CAN3/FD_THCM1_0x182 ==
  BSCP_outputs : Inport  OutDataTypeStr=Bus: BSCP_outputs
  BOUTP_outputs : Inport  Port=2  OutDataTypeStr=Bus: BOUTP_outputs
  BatteryMode : Subsystem
  CCUACLampSts : Subsystem
  CCUACMaxLampSts : Subsystem
  CCUAutoLampSts : Subsystem
  CCUAutoMidLampSts : Subsystem
  CCUDispalyRequest : Subsystem
  CCUEcoSts : Subsystem
  CCUFrtOnOffLampSts : Subsystem
  CCUHEATMaxLampSts : Subsystem
  CCURrOnOffLampSts : Subsystem
  CCUSyncLampSts : Subsystem
  CabinMode : Subsystem
  EDriveMode : Subsystem
  FDAGSCmd : Subsystem
  FDRecyAutoCmd : Subsystem
  FrCoolantflow : Subsystem
  FrCoolanttemp : Subsystem
  Ground{,1..17} (18 alike) : Ground
  HPThermalRecoveryReq : Subsystem
  RrCoolantflow : Subsystem
  RrCoolanttemp : Subsystem
  bus_creator : BusCreator  Inputs=37  OutDataTypeStr=Bus: DT_CAN3_SG_FD_THCM1  NonVirtualBus=on
  bus_selector : BusSelector  OutputSignals=VOUTP_BatteryMode_enum
  bus_selector1 : BusSelector  OutputSignals=VOUTP_CCUACLampSts_flg
  bus_selector10 : BusSelector  OutputSignals=VOUTP_sigAmbAirT_C
  bus_selector11 : BusSelector  OutputSignals=VOUTP_sigCbnAirT_C
  bus_selector12 : BusSelector  OutputSignals=VOUTP_sigCbnSolarLeft_W
  bus_selector13 : BusSelector  OutputSignals=VOUTP_sigCbnSolarRight_W
  bus_selector14 : BusSelector  OutputSignals=VOUTP_sigClntTHvBattOut_C
  bus_selector15 : BusSelector  OutputSignals=VOUTP_sigRecircSt_flg
  bus_selector16 : BusSelector  OutputSignals=VOUTP_sigSetTempZon1St_C
  bus_selector17 : BusSelector  OutputSignals=VOUTP_sigSetTempZon2St_C
  bus_selector18 : BusSelector  OutputSignals=VOUTP_sigWindDirZon1St_enum
  bus_selector2 : BusSelector  OutputSignals=VOUTP_CCUACMaxLampSts_flg
  bus_selector3 : BusSelector  OutputSignals=VOUTP_CCUAutoLampSts_flg
  bus_selector4 : BusSelector  OutputSignals=VOUTP_CCUSyncLampSts_flg
  bus_selector5 : BusSelector  OutputSignals=VOUTP_CabinMode_enum
  bus_selector6 : BusSelector  OutputSignals=VOUTP_EDriveMode_enum
  bus_selector7 : BusSelector  OutputSignals=VOUTP_FDAGSCmd_enum
  bus_selector8 : BusSelector  OutputSignals=VOUTP_FDRecyAutoCmd_enum
  bus_selector9 : BusSelector  OutputSignals=VOUTP_sigAirIntenZon1St_enum
  sigAirIntenZon1St : Subsystem
  sigAirIntenZon3St : Subsystem
  sigAmbAirT : Subsystem
  sigCbnAirT : Subsystem
  sigCbnPTCPwrAct : Subsystem
  sigCbnSolarLeft : Subsystem
  sigCbnSolarRight : Subsystem
  sigClmtCmprPwrAct : Subsystem
  sigClntTHvBattOut : Subsystem
  sigDfrstSt : Subsystem
  sigHvacSt : Subsystem
  sigRecircSt : Subsystem
  sigSetTempZon1St : Subsystem
  sigSetTempZon2St : Subsystem
  sigSetTempZon3St : Subsystem
  sigWindDirZon1St : Subsystem
  sigWindDirZon3St : Subsystem
  FD_THCM1 : Outport
  wires:
  BSCP_outputs/1 -> [BSCP_outputs]
  BOUTP_outputs/1 -> [BOUTP_outputs]
  [CAN3_BatteryMode] -> bus_creator/1  "CAN3_BatteryMode"
  [CAN3_CCU_ACLampSts] -> bus_creator/2  "CAN3_CCU_ACLampSts"
  [CAN3_CCU_ACMaxLampSts] -> bus_creator/3  "CAN3_CCU_ACMaxLampSts"
  [CAN3_CCU_AutoLampSts] -> bus_creator/4  "CAN3_CCU_AutoLampSts"
  [CAN3_CCU_AutoMidLampSts] -> bus_creator/5  "CAN3_CCU_AutoMidLampSts"
  [CAN3_CCU_Dispaly_Request] -> bus_creator/6  "CAN3_CCU_Dispaly_Request"
  [CAN3_CCU_EcoSts] -> bus_creator/7  "CAN3_CCU_EcoSts"
  [CAN3_CCU_FrtOnOffLampSts] -> bus_creator/8  "CAN3_CCU_FrtOnOffLampSts"
  [CAN3_CCU_HEATMaxLampSts] -> bus_creator/9  "CAN3_CCU_HEATMaxLampSts"
  [CAN3_CCU_RrOnOffLampSts] -> bus_creator/10  "CAN3_CCU_RrOnOffLampSts"
  [CAN3_CCU_SyncLampSts] -> bus_creator/11  "CAN3_CCU_SyncLampSts"
  [CAN3_CabinMode] -> bus_creator/12  "CAN3_CabinMode"
  [CAN3_EDriveMode] -> bus_creator/13  "CAN3_EDriveMode"
  [CAN3_FD_AGS_Cmd] -> bus_creator/14  "CAN3_FD_AGS_Cmd"
  [CAN3_FD_RecyAuto_Cmd] -> bus_creator/15  "CAN3_FD_RecyAuto_Cmd"
  [CAN3_Fr_Coolantflow] -> bus_creator/16  "CAN3_Fr_Coolantflow"
  [CAN3_Fr_Coolanttemp] -> bus_creator/17  "CAN3_Fr_Coolanttemp"
  [CAN3_HPThermalRecoveryReq] -> bus_creator/18  "CAN3_HPThermalRecoveryReq"
  [CAN3_Rr_Coolantflow] -> bus_creator/19  "CAN3_Rr_Coolantflow"
  [CAN3_Rr_Coolanttemp] -> bus_creator/20  "CAN3_Rr_Coolanttemp"
  [CAN3_sigAirIntenZon1St] -> bus_creator/21  "CAN3_sigAirIntenZon1St"
  [CAN3_sigAirIntenZon3St] -> bus_creator/22  "CAN3_sigAirIntenZon3St"
  [CAN3_sigAmbAirT] -> bus_creator/23  "CAN3_sigAmbAirT"
  [CAN3_sigCbnAirT] -> bus_creator/24  "CAN3_sigCbnAirT"
  [CAN3_sigCbnPTCPwrAct] -> bus_creator/25  "CAN3_sigCbnPTCPwrAct"
  [CAN3_sigCbnSolarLeft] -> bus_creator/26  "CAN3_sigCbnSolarLeft"
  [CAN3_sigCbnSolarRight] -> bus_creator/27  "CAN3_sigCbnSolarRight"
  [CAN3_sigClmtCmprPwrAct] -> bus_creator/28  "CAN3_sigClmtCmprPwrAct"
  [CAN3_sigClntTHvBattOut] -> bus_creator/29  "CAN3_sigClntTHvBattOut"
  [CAN3_sigDfrstSt] -> bus_creator/30  "CAN3_sigDfrstSt"
  [CAN3_sigHvacSt] -> bus_creator/31  "CAN3_sigHvacSt"
  [CAN3_sigRecircSt] -> bus_creator/32  "CAN3_sigRecircSt"
  [CAN3_sigSetTempZon1St] -> bus_creator/33  "CAN3_sigSetTempZon1St"
  [CAN3_sigSetTempZon2St] -> bus_creator/34  "CAN3_sigSetTempZon2St"
  [CAN3_sigSetTempZon3St] -> bus_creator/35  "CAN3_sigSetTempZon3St"
  [CAN3_sigWindDirZon1St] -> bus_creator/36  "CAN3_sigWindDirZon1St"
  [CAN3_sigWindDirZon3St] -> bus_creator/37  "CAN3_sigWindDirZon3St"
  bus_creator/1 -> FD_THCM1/1
  BatteryMode/1(CAN3_BatteryMode) -> [CAN3_BatteryMode]
  CCUACLampSts/1(CAN3_CCU_ACLampSts) -> [CAN3_CCU_ACLampSts]
  CCUACMaxLampSts/1(CAN3_CCU_ACMaxLampSts) -> [CAN3_CCU_ACMaxLampSts]
  CCUAutoLampSts/1(CAN3_CCU_AutoLampSts) -> [CAN3_CCU_AutoLampSts]
  CCUAutoMidLampSts/1(CAN3_CCU_AutoMidLampSts) -> [CAN3_CCU_AutoMidLampSts]
  CCUDispalyRequest/1(CAN3_CCU_Dispaly_Request) -> [CAN3_CCU_Dispaly_Request]
  CCUEcoSts/1(CAN3_CCU_EcoSts) -> [CAN3_CCU_EcoSts]
  CCUFrtOnOffLampSts/1(CAN3_CCU_FrtOnOffLampSts) -> [CAN3_CCU_FrtOnOffLampSts]
  CCUHEATMaxLampSts/1(CAN3_CCU_HEATMaxLampSts) -> [CAN3_CCU_HEATMaxLampSts]
  CCURrOnOffLampSts/1(CAN3_CCU_RrOnOffLampSts) -> [CAN3_CCU_RrOnOffLampSts]
  CCUSyncLampSts/1(CAN3_CCU_SyncLampSts) -> [CAN3_CCU_SyncLampSts]
  CabinMode/1(CAN3_CabinMode) -> [CAN3_CabinMode]
  EDriveMode/1(CAN3_EDriveMode) -> [CAN3_EDriveMode]
  FDAGSCmd/1(CAN3_FD_AGS_Cmd) -> [CAN3_FD_AGS_Cmd]
  FDRecyAutoCmd/1(CAN3_FD_RecyAuto_Cmd) -> [CAN3_FD_RecyAuto_Cmd]
  FrCoolantflow/1(CAN3_Fr_Coolantflow) -> [CAN3_Fr_Coolantflow]
  FrCoolanttemp/1(CAN3_Fr_Coolanttemp) -> [CAN3_Fr_Coolanttemp]
  HPThermalRecoveryReq/1(CAN3_HPThermalRecoveryReq) -> [CAN3_HPThermalRecoveryReq]
  RrCoolantflow/1(CAN3_Rr_Coolantflow) -> [CAN3_Rr_Coolantflow]
  RrCoolanttemp/1(CAN3_Rr_Coolanttemp) -> [CAN3_Rr_Coolanttemp]
  sigAirIntenZon1St/1(CAN3_sigAirIntenZon1St) -> [CAN3_sigAirIntenZon1St]
  sigAirIntenZon3St/1(CAN3_sigAirIntenZon3St) -> [CAN3_sigAirIntenZon3St]
  sigAmbAirT/1(CAN3_sigAmbAirT) -> [CAN3_sigAmbAirT]
  sigCbnAirT/1(CAN3_sigCbnAirT) -> [CAN3_sigCbnAirT]
  sigCbnPTCPwrAct/1(CAN3_sigCbnPTCPwrAct) -> [CAN3_sigCbnPTCPwrAct]
  sigCbnSolarLeft/1(CAN3_sigCbnSolarLeft) -> [CAN3_sigCbnSolarLeft]
  sigCbnSolarRight/1(CAN3_sigCbnSolarRight) -> [CAN3_sigCbnSolarRight]
  sigClmtCmprPwrAct/1(CAN3_sigClmtCmprPwrAct) -> [CAN3_sigClmtCmprPwrAct]
  sigClntTHvBattOut/1(CAN3_sigClntTHvBattOut) -> [CAN3_sigClntTHvBattOut]
  sigDfrstSt/1(CAN3_sigDfrstSt) -> [CAN3_sigDfrstSt]
  sigHvacSt/1(CAN3_sigHvacSt) -> [CAN3_sigHvacSt]
  sigRecircSt/1(CAN3_sigRecircSt) -> [CAN3_sigRecircSt]
  sigSetTempZon1St/1(CAN3_sigSetTempZon1St) -> [CAN3_sigSetTempZon1St]
  sigSetTempZon2St/1(CAN3_sigSetTempZon2St) -> [CAN3_sigSetTempZon2St]
  sigSetTempZon3St/1(CAN3_sigSetTempZon3St) -> [CAN3_sigSetTempZon3St]
  sigWindDirZon1St/1(CAN3_sigWindDirZon1St) -> [CAN3_sigWindDirZon1St]
  sigWindDirZon3St/1(CAN3_sigWindDirZon3St) -> [CAN3_sigWindDirZon3St]
  bus_selector/1 -> BatteryMode/1(BatteryMode)  "<VOUTP_BatteryMode_enum>"
  [BOUTP_outputs] -> bus_selector/1
  bus_selector1/1 -> CCUACLampSts/1(CCUACLampSts)  "<VOUTP_CCUACLampSts_flg>"
  [BOUTP_outputs] -> bus_selector1/1
  bus_selector2/1 -> CCUACMaxLampSts/1(CCUACMaxLampSts)  "<VOUTP_CCUACMaxLampSts_flg>"
  [BOUTP_outputs] -> bus_selector2/1
  bus_selector3/1 -> CCUAutoLampSts/1(CCUAutoLampSts)  "<VOUTP_CCUAutoLampSts_flg>"
  [BOUTP_outputs] -> bus_selector3/1
  Ground/1 -> CCUAutoMidLampSts/1(CCUAutoMidLampSts)
  Ground1/1 -> CCUDispalyRequest/1(CCUDispalyRequest)
  Ground2/1 -> CCUEcoSts/1(CCUEcoSts)
  Ground3/1 -> CCUFrtOnOffLampSts/1(CCUFrtOnOffLampSts)
  Ground4/1 -> CCUHEATMaxLampSts/1(CCUHEATMaxLampSts)
  Ground5/1 -> CCURrOnOffLampSts/1(CCURrOnOffLampSts)
  bus_selector4/1 -> CCUSyncLampSts/1(CCUSyncLampSts)  "<VOUTP_CCUSyncLampSts_flg>"
  [BOUTP_outputs] -> bus_selector4/1
  bus_selector5/1 -> CabinMode/1(CabinMode)  "<VOUTP_CabinMode_enum>"
  [BOUTP_outputs] -> bus_selector5/1
  bus_selector6/1 -> EDriveMode/1(EDriveMode)  "<VOUTP_EDriveMode_enum>"
  [BOUTP_outputs] -> bus_selector6/1
  bus_selector7/1 -> FDAGSCmd/1(FDAGSCmd)  "<VOUTP_FDAGSCmd_enum>"
  [BOUTP_outputs] -> bus_selector7/1
  bus_selector8/1 -> FDRecyAutoCmd/1(FDRecyAutoCmd)  "<VOUTP_FDRecyAutoCmd_enum>"
  [BOUTP_outputs] -> bus_selector8/1
  Ground6/1 -> FrCoolantflow/1(FrCoolantflow)
  Ground7/1 -> FrCoolanttemp/1(FrCoolanttemp)
  Ground8/1 -> HPThermalRecoveryReq/1(HPThermalRecoveryReq)
  Ground9/1 -> RrCoolantflow/1(RrCoolantflow)
  Ground10/1 -> RrCoolanttemp/1(RrCoolanttemp)
  bus_selector9/1 -> sigAirIntenZon1St/1(sigAirIntenZon1St)  "<VOUTP_sigAirIntenZon1St_enum>"
  [BOUTP_outputs] -> bus_selector9/1
  Ground11/1 -> sigAirIntenZon3St/1(sigAirIntenZon3St)
  bus_selector10/1 -> sigAmbAirT/1(sigAmbAirT)  "<VOUTP_sigAmbAirT_C>"
  [BOUTP_outputs] -> bus_selector10/1
  bus_selector11/1 -> sigCbnAirT/1(sigCbnAirT)  "<VOUTP_sigCbnAirT_C>"
  [BOUTP_outputs] -> bus_selector11/1
  Ground12/1 -> sigCbnPTCPwrAct/1(sigCbnPTCPwrAct)
  bus_selector12/1 -> sigCbnSolarLeft/1(sigCbnSolarLeft)  "<VOUTP_sigCbnSolarLeft_W>"
  [BOUTP_outputs] -> bus_selector12/1
  bus_selector13/1 -> sigCbnSolarRight/1(sigCbnSolarRight)  "<VOUTP_sigCbnSolarRight_W>"
  [BOUTP_outputs] -> bus_selector13/1
  Ground13/1 -> sigClmtCmprPwrAct/1(sigClmtCmprPwrAct)
  bus_selector14/1 -> sigClntTHvBattOut/1(sigClntTHvBattOut)  "<VOUTP_sigClntTHvBattOut_C>"
  [BOUTP_outputs] -> bus_selector14/1
  Ground14/1 -> sigDfrstSt/1(sigDfrstSt)
  Ground15/1 -> sigHvacSt/1(sigHvacSt)
  bus_selector15/1 -> sigRecircSt/1(sigRecircSt)  "<VOUTP_sigRecircSt_flg>"
  [BOUTP_outputs] -> bus_selector15/1
  bus_selector16/1 -> sigSetTempZon1St/1(sigSetTempZon1St)  "<VOUTP_sigSetTempZon1St_C>"
  [BOUTP_outputs] -> bus_selector16/1
  bus_selector17/1 -> sigSetTempZon2St/1(sigSetTempZon2St)  "<VOUTP_sigSetTempZon2St_C>"
  [BOUTP_outputs] -> bus_selector17/1
  Ground16/1 -> sigSetTempZon3St/1(sigSetTempZon3St)
  bus_selector18/1 -> sigWindDirZon1St/1(sigWindDirZon1St)  "<VOUTP_sigWindDirZon1St_enum>"
  [BOUTP_outputs] -> bus_selector18/1
  Ground17/1 -> sigWindDirZon3St/1(sigWindDirZon3St)
